simulink model "sysID_1"  (R2024a)
settings: Solver=VariableStepAuto  StartTime=0.0  StopTime=T + Ttrans - Ts  RelTol=1e-3
values from neighbouring files (symbols this model uses):
  K = db2mag(-8.5)    [systemID_GyroPost.m]
undefined symbols (not defined in the file or in its folder): N, Q1e, T, Ts, w1e, w2e
libraries: cstblocks x1
settings Model: Creator=dunni  LastModifiedBy=dunni

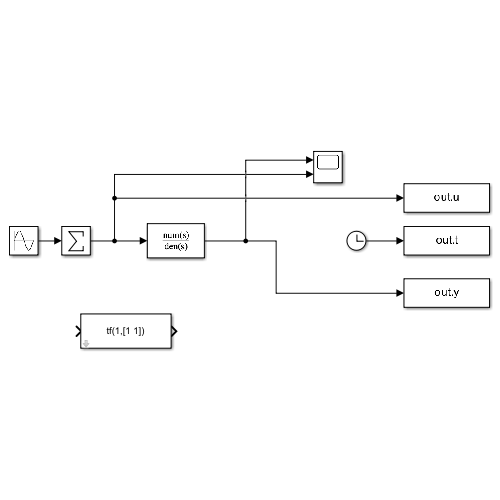
[thumbnail: Simulink's stored preview of the top-level diagram]
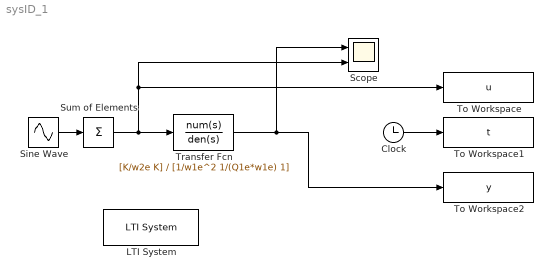
== system sysID_1 ==
  Clock : Clock
  LTI System : cstblocks/LTI System  sys=tf(1,[1 1])  IC=[]  PadeOrder=0
  Scope : Scope  NumInputPorts=2
  Sine Wave : Sin  Frequency=(1:N)*2*pi/T  Phase=rand(N,1)*2*pi  SampleTime=0
  Sum of Elements : Sum  Inputs=+
  To Workspace : ToWorkspace  VariableName=u  SampleTime=Ts
      settings: MaxDataPoints=T/Ts
  To Workspace1 : ToWorkspace  VariableName=t  SampleTime=Ts
      settings: MaxDataPoints=T/Ts
  To Workspace2 : ToWorkspace  VariableName=y  SampleTime=Ts
      settings: MaxDataPoints=T/Ts
  Transfer Fcn : TransferFcn  Numerator=[K/w2e K]  Denominator=[1/w1e^2 1/(Q1e*w1e) 1]
  wires:
  Sine Wave/1 -> Sum of Elements/1
  Clock/1 -> To Workspace1/1
  Sum of Elements/1 -> Transfer Fcn/1, To Workspace/1, Scope/2
  Transfer Fcn/1 -> Scope/1, To Workspace2/1
